simulink model "Controller"  (R2023b)
settings: Solver=VariableStepAuto  StartTime=0.0  StopTime=10.0  RelTol=1e-3
model workspace (MAT data in the model file):
  J = 7
  K = 1.4
  K1 = 0.02
  L = 0.1
  R = 0.4
  TL = 5
  Vin = 12

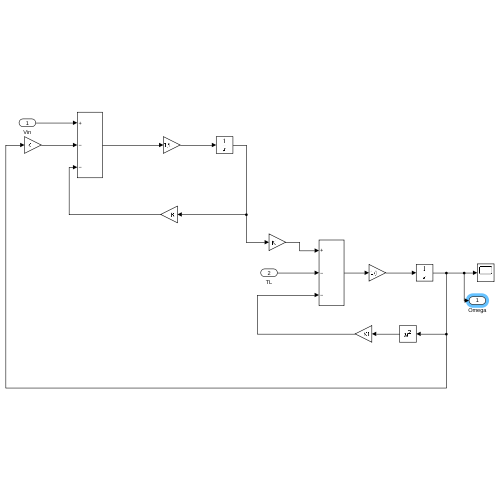
[thumbnail: Simulink's stored preview of the top-level diagram]
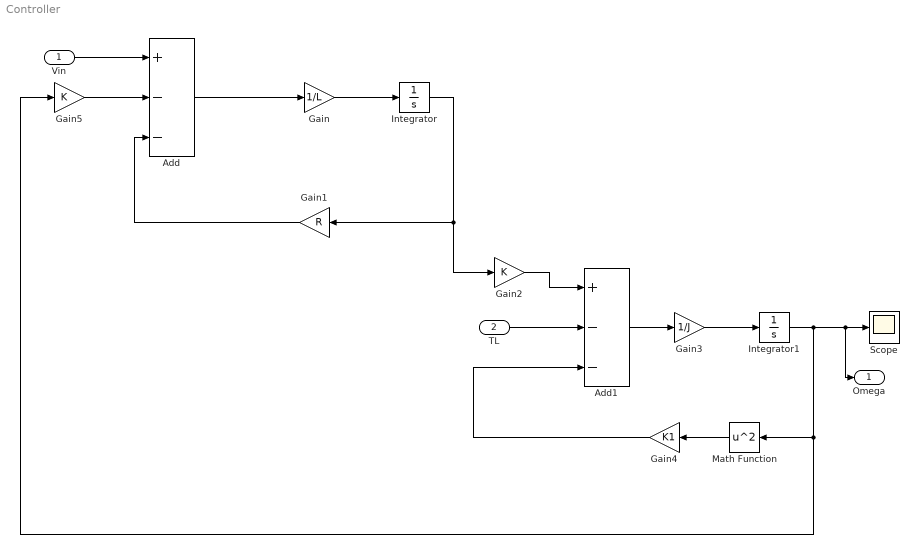
== system Controller ==
  Vin : Inport
  TL : Inport  Port=2
  Add : Sum  Inputs=+--
  Add1 : Sum  Inputs=+--
  Gain : Gain  Gain=1/L
  Gain1 : Gain  Gain=R
  Gain2 : Gain  Gain=K
  Gain3 : Gain  Gain=1/J
  Gain4 : Gain  Gain=K1
  Gain5 : Gain  Gain=K
  Integrator : Integrator
  Integrator1 : Integrator
  Math Function : Math  Operator=square
  Scope : Scope
  Omega : Outport
  wires:
  Vin/1 -> Add/1
  Add/1 -> Gain/1
  Gain/1 -> Integrator/1
  Integrator/1 -> Gain1/1, Gain2/1
  Gain1/1 -> Add/3
  Gain2/1 -> Add1/1
  TL/1 -> Add1/2
  Add1/1 -> Gain3/1
  Gain3/1 -> Integrator1/1
  Integrator1/1 -> Omega/1, Scope/1, Math Function/1, Gain5/1
  Gain4/1 -> Add1/3
  Math Function/1 -> Gain4/1
  Gain5/1 -> Add/2
